simulink subsystem "RegulatorRobustDigital_SubSystem"  (R2020b)
settings: Solver=VariableStepAuto  StartTime=0.0  StopTime=10.0  RelTol=1e-3
values from neighbouring files (symbols this model uses):
  C = [1,0]    [StateSpaceControllerNominalCont.m]    (also in StateSpaceControllerNominalDigital.m; StateSpaceControllerNominalDirectDigital.m; StateSpaceControllerRobustCont.m; StateSpaceControllerRobustDigital.m)
  Gamma0 = [Gamma2 - L*Gamma1,(Phi22 - L*Phi12)*L+Phi21-L*Phi11]    [StateSpaceControllerNominalDirectDigital.m]    (also in StateSpaceControllerRobustDirectDigital.m)
  H0 = T*[zeros(pOutput,size(Phi,1) - pOutput);eye(size(Phi,1) - pOutput)]    [StateSpaceControllerNominalDirectDigital.m]    (also in StateSpaceControllerRobustDirectDigital.m)
  J0 = T*[zeros(pOutput,mInput),eye(pOutput);         zeros(size(Phi,1) - pOutput,mInput),L]    [StateSpaceControllerNominalDirectDigital.m]    (also in StateSpaceControllerRobustDirectDigital.m)
  Ke = Ke_4    [StateSpaceControllerRobustCont.m]    (also in StateSpaceControllerRobustDigital.m; StateSpaceControllerRobustDirectDigital.m = place(Phie,Gammae,p))
  Nu = reshape(Nu,[],1)    [StateSpaceControllerNominalCont.m]    (also in StateSpaceControllerNominalDigital.m; StateSpaceControllerNominalDirectDigital.m; StateSpaceControllerRobustCont.m; StateSpaceControllerRobustDigital.m)
  Nx = reshape(Nx,[],1)    [StateSpaceControllerNominalCont.m]    (also in StateSpaceControllerNominalDigital.m; StateSpaceControllerNominalDirectDigital.m; StateSpaceControllerRobustCont.m; StateSpaceControllerRobustDigital.m)
  Phi0 = Phi22 - L*Phi12    [StateSpaceControllerNominalDirectDigital.m]    (also in StateSpaceControllerRobustDirectDigital.m)
  Ts = T2    (= 0.01)    [PIDAntiWindupDigital.m]    (also in PIDDigital.m = 0.001; StateSpaceControllerNominalCont.m = 0.001; StateSpaceControllerNominalDigital.m = 0.001; StateSpaceControllerNominalDirectDigital.m = 0.05)
undefined symbols (not defined in the file or in its folder): DiscIntNeverNeededParam
settings Model: Creator=umberto  LastModifiedBy=umbe

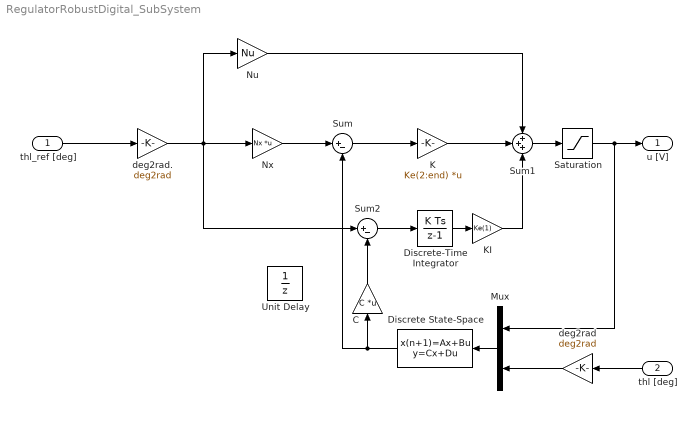
== system RegulatorRobustDigital_SubSystem ==
  thl_ref [deg] : Inport
  thl [deg] : Inport  Port=2
  C : Gain  Gain=C  Multiplication=Matrix(K*u)
  Discrete State-Space : DiscreteStateSpace  A=Phi0  B=Gamma0  C=H0  D=J0  SampleTime=Ts
  Discrete-Time Integrator : DiscreteIntegrator  SampleTime=Ts  ICPrevOutput=DiscIntNeverNeededParam  ICPrevScaledInput=DiscIntNeverNeededParam
  K : Gain  Gain=Ke(2:end)  Multiplication=Matrix(K*u)
  KI : Gain  Gain=Ke(1)
  Mux : Mux  Inputs=2
  Nu : Gain  Gain=Nu
  Nx : Gain  Gain=Nx  Multiplication=Matrix(K*u)
  Saturation : Saturate  UpperLimit=10  LowerLimit=-10
  Sum : Sum  Inputs=|+-
  Sum1 : Sum  Inputs=+++
  Sum2 : Sum  Inputs=|+-
  Unit Delay : UnitDelay  SampleTime=Ts  HasFrameUpgradeWarning=on
  deg2rad : Gain  Gain=deg2rad
  deg2rad. : Gain  Gain=deg2rad
  u [V] : Outport
  wires:
  deg2rad/1 -> Mux/2
  thl [deg]/1 -> deg2rad/1
  thl_ref [deg]/1 -> deg2rad./1
  deg2rad./1 -> Sum2/1, Nu/1, Nx/1
  Nx/1 -> Sum/1
  Sum/1 -> K/1
  K/1 -> Sum1/2
  Nu/1 -> Sum1/1
  Sum1/1 -> Saturation/1
  Saturation/1 -> u [V]/1, Mux/1
  C/1 -> Sum2/2
  KI/1 -> Sum1/3
  Mux/1 -> Discrete State-Space/1
  Discrete State-Space/1 -> C/1, Sum/2
  Sum2/1 -> Discrete-Time Integrator/1
  Discrete-Time Integrator/1 -> KI/1
